simulink model "A02_L5_1_2015"  (R2015b)
settings: Solver=ode45  StartTime=0.0  StopTime=0.04  RelTol=1e-3
values from neighbouring files (symbols this model uses):
  alfa = 3+a    (= 7)    [A04_L5_script.m]
  beta = 1+0.25*b    (= 1.5)    [A04_L5_script.m]
settings Model: Creator=User  LastModifiedBy=Ana
settings DataIOCC: SaveFormat=Array
settings DebuggingCC: SolverPrmCheckMsg=warning  AllowSymbolicDim=on
settings HardwareCC: ProdBitPerPointer=32  ProdLargestAtomicFloat=None  ProdIntDivRoundTo=Undefined  ProdEndianess=Unspecified  ProdWordSize=32  ProdHWDeviceType=32-bit Generic
settings GRTTargetCC: GeneratePreprocessorConditionals=Disable all
settings ConfigComp: CovModelRefEnable=Off  CovSFcnEnable=off

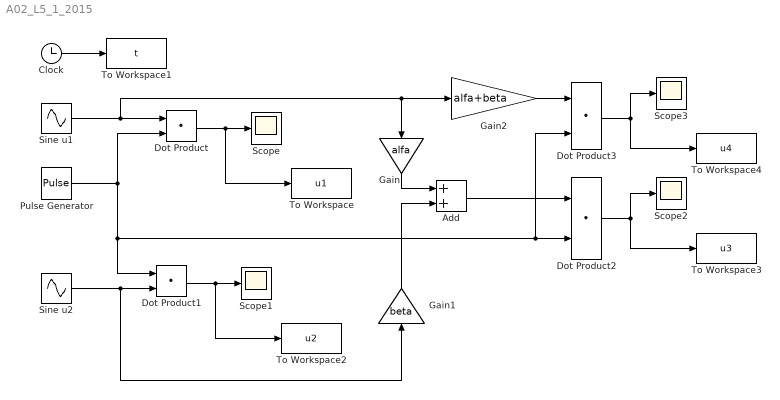
== system A02_L5_1_2015 ==
  Add : Sum
  Clock : Clock
  Dot Product{,1..3} (4 alike) : DotProduct  InputSameDT=on  OutDataTypeStr=Inherit: Inherit via internal rule
  Gain : Gain  Gain=alfa
  Gain1 : Gain  Gain=beta
  Gain2 : Gain  Gain=alfa+beta
  Pulse Generator : DiscretePulseGenerator  PulseType=Time based  Period=1/400  PulseWidth=0.1
  Scope{,1..3} (4 alike) : Scope
  Sine u1 : Sin  Amplitude=70  Frequency=300*pi  Phase=0.23  SampleTime=0
  Sine u2 : Sin  Amplitude=70  Frequency=2700*pi  Phase=0.23  SampleTime=0
  To Workspace : ToWorkspace  VariableName=u1  SampleTime=-1
  To Workspace1 : ToWorkspace  VariableName=t  SampleTime=-1
  To Workspace2 : ToWorkspace  VariableName=u2  SampleTime=-1
  To Workspace3 : ToWorkspace  VariableName=u3  SampleTime=-1
  To Workspace4 : ToWorkspace  VariableName=u4  SampleTime=-1
  wires:
  Clock/1 -> To Workspace1/1
  Sine u1/1 -> Gain2/1, Gain/1, Dot Product/1
  Dot Product/1 -> To Workspace/1, Scope/1
  Sine u2/1 -> Dot Product1/2, Gain1/1
  Dot Product1/1 -> To Workspace2/1, Scope1/1
  Gain/1 -> Add/1
  Gain1/1 -> Add/2
  Add/1 -> Dot Product2/1
  Pulse Generator/1 -> Dot Product3/2, Dot Product2/2, Dot Product1/1, Dot Product/2
  Dot Product2/1 -> Scope2/1, To Workspace3/1
  Gain2/1 -> Dot Product3/1
  Dot Product3/1 -> To Workspace4/1, Scope3/1
